simulink model "sl_quadrotorDynamics"  (R2024b)
settings: Solver=VariableStepAuto  StartTime=0.0  StopTime=50  MaxStep=0.1  RelTol=1e-3  EnableMultiTasking=on
InitFcn:
  | % load parameters of the default quadrotor
  | disp('Quadrotor parameters loaded by InitFcn')
  | mdl_quadrotor
libraries: simulink x2, roblocks x1
settings Model: Creator=corkep  LastModifiedBy=mejiasal@qut.edu.au
settings SolverCC: ZeroCrossAlgorithm=Adaptive  AlgebraicLoopSolver=TrustRegion
settings DataIOCC: LimitDataPoints=on  SaveFormat=Array  ReturnWorkspaceOutputs=off
settings OptimizationCC: BlockReduction=off  BooleanDataType=off  ReuseModelBlockBuffer=off  LifeSpan=inf
settings DebuggingCC: SaveWithParameterizedLinksMsg=none  MergeDetectMultiDrivingBlocksExec=none  SignalResolutionControl=TryResolveAllWithWarning  MaskedZcDiagnostic=none  IgnoredZcDiagnostic=none  UnconnectedInputMsg=warning  UnconnectedOutputMsg=warning  UnconnectedLineMsg=warning  SFUnexpectedBacktrackingDiag=warning  SFNoUnconditionalDefaultTransitionDiag=warning  SFExecutionAtInitializationDiag=none  ArithmeticOperatorsInVariantConditions=warning
settings HardwareCC: ProdBitPerPointer=32  ProdBitPerSizeT=32  ProdBitPerPtrDiffT=32  ProdLargestAtomicFloat=None  ProdIntDivRoundTo=Undefined  ProdEndianess=Unspecified  ProdWordSize=32  ProdHWDeviceType=32-bit Generic  TargetUnknown=on
settings ModelReferenceCC: EnableRefExpFcnMdlSchedulingChecks=on  PropagateSignalLabelsOutOfModel=off
settings SFSimCC: SimUseLocalCustomCode=off  CustomCodeUndefinedFunction=UseInterfaceOnly
settings RTWCC: RTWUseLocalCustomCode=off  GPUComputeCapability=3.5
settings CodeAppCC: StateflowObjectComments=on
settings GRTTargetCC: TargetLangStandard=C89/C90 (ANSI)
settings ConfigComp: CovMetricSettings=dw  CovSaveCumulativeToWorkspaceVar=on  CovSaveSingleToWorkspaceVar=on  CovExternalEMLEnable=off  CovSFcnEnable=off

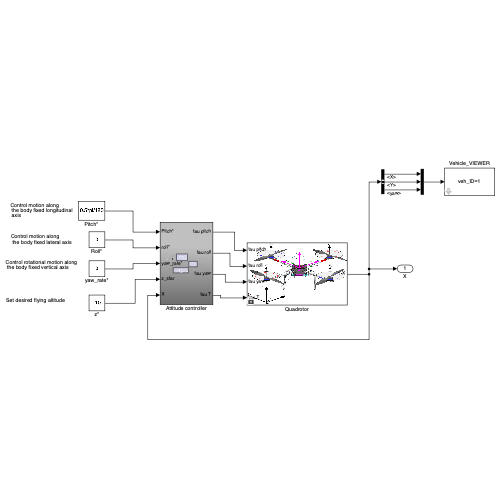
[thumbnail: Simulink's stored preview of the top-level diagram]
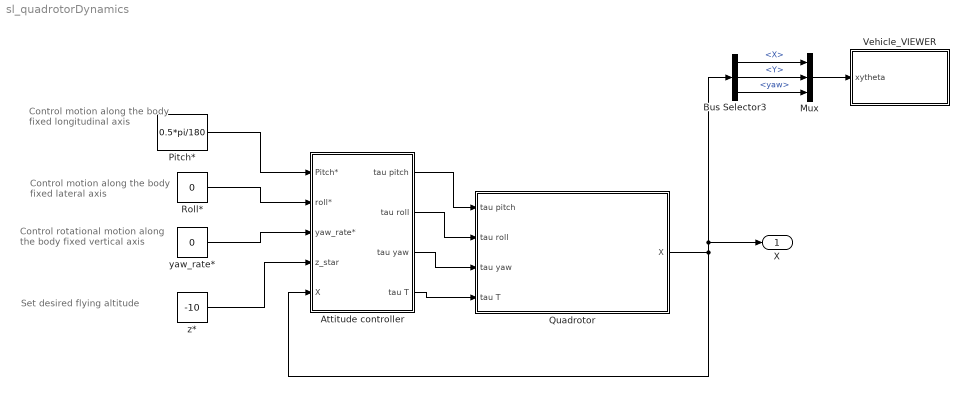
== system sl_quadrotorDynamics ==
  note: Control motion along
      |  the body fixed lateral axis
  note: Control motion along
      |  the body fixed longitudinal
      |  axis
  note: Control rotational motion along
      |  the body fixed vertical axis
  note: Set desired flying altitude
  Attitude controller : Subsystem
  Bus Selector3 : BusSelector  OutputSignals=X,Y,yaw
  Mux : Mux  Inputs=3
  Pitch* : Constant  Value=0.5*pi/180
  Quadrotor : Subsystem
      mask Display: image('quadrotor.png');
  Roll* : Constant  Value=0
  Vehicle_VIEWER : Subsystem  mask{wp_mat=[-100, 100;-100, 100]', veh_ID_num=1, veh_init_xytheta=[0 0 0], Ts=0.1}
      mask prompts: wp_mat "Waypoint matrix for arena [x_col, y_col, z_col, angle_col] (m, deg)"; veh_ID_num "Vehicle ID number"; veh_init_xytheta "Initial pose [x,y, psi]"; Ts "Sample time for updating animation (secs)"
      mask TypeOptions veh_ID_num: 1 | 2 | 3 | 4
      mask DialogControl Control2 Prompt: Animate simulation of Robot
      mask Display: fprintf('veh_ID=%d',veh_ID_num);
  yaw_rate* : Constant  Value=0
  z* : Constant  Value=-10
  X : Outport
  wires:
  Bus Selector3/1 -> Mux/1  "<X>"
  Bus Selector3/2 -> Mux/2  "<Y>"
  Bus Selector3/3 -> Mux/3  "<yaw>"
  Mux/1 -> Vehicle_VIEWER/1(xytheta)
  Roll*/1 -> Attitude controller/2(roll*)
  z*/1 -> Attitude controller/4(z_star)
  Pitch*/1 -> Attitude controller/1(Pitch*)
  yaw_rate*/1 -> Attitude controller/3(yaw_rate*)
  Quadrotor/1(X) -> X/1, Bus Selector3/1, Attitude controller/5(X)
  Attitude controller/1(tau pitch) -> Quadrotor/1(tau pitch)
  Attitude controller/2(tau roll) -> Quadrotor/2(tau roll)
  Attitude controller/3(tau yaw) -> Quadrotor/3(tau yaw)
  Attitude controller/4(tau T) -> Quadrotor/4(tau T)

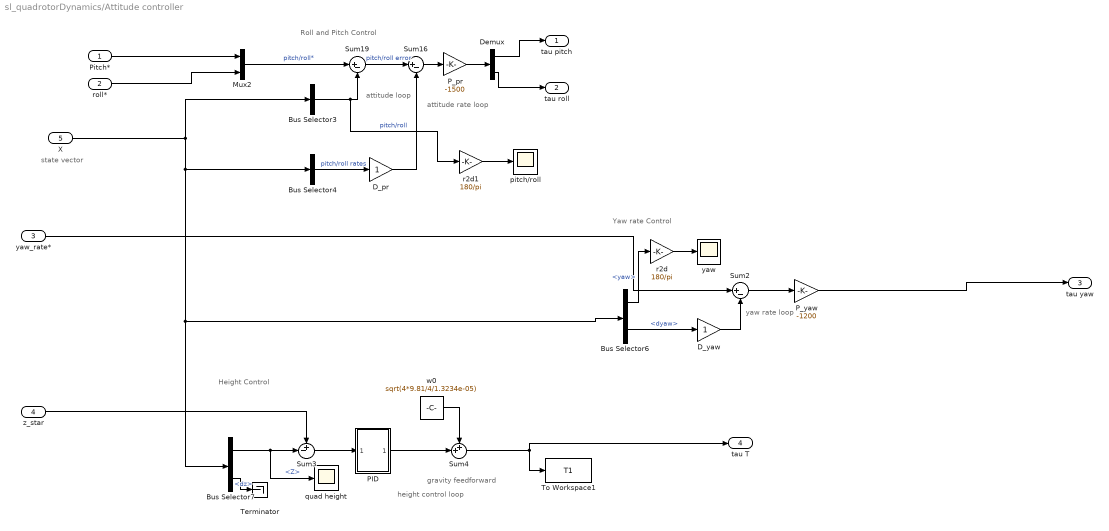
== system sl_quadrotorDynamics/Attitude controller ==
  note: Height Control
  note: Yaw rate Control
  note: Roll and Pitch Control
  note: state vector
  note: gravity feedforward
  note: attitude rate
      | loop
  note: height control
      | loop
  note: attitude
      | loop
  note: yaw rate
      | loop
  Pitch* : Inport
  roll* : Inport  Port=2
  yaw_rate* : Inport  Port=3
  z_star : Inport  Port=4
  X : Inport  Port=5
  Bus Selector3 : BusSelector  OutputSignals=pitch,roll  OutputAsBus=on
  Bus Selector4 : BusSelector  OutputSignals=dpitch,droll  OutputAsBus=on
  Bus Selector6 : BusSelector  OutputSignals=yaw,dyaw
  Bus Selector7 : BusSelector  OutputSignals=Z,dz
  D_pr : Gain
  D_yaw : Gain
  Demux : Demux  Outputs=2
  Mux2 : Mux  Inputs=2
  PID : Subsystem
  P_pr : Gain  Gain=-1500
  P_yaw : Gain  Gain=-1200
  Sum16 : Sum  Inputs=|+-
  Sum19 : Sum  Inputs=|+-
  Sum2 : Sum  Inputs=|+-
  Sum3 : Sum  Inputs=+-|
  Sum4 : Sum  Inputs=++|
  Terminator : Terminator
  To Workspace1 : ToWorkspace  VariableName=T1  SampleTime=-1
  pitch/roll : Scope
  quad height : Scope
  r2d : Gain  Gain=180/pi
  r2d1 : Gain  Gain=180/pi
  w0 : Constant  Value=sqrt(4*9.81/4/1.3234e-05)  SampleTime=0
  yaw : Scope
  tau pitch : Outport  VectorParamsAs1DForOutWhenUnconnected=off
  tau roll : Outport  Port=2  VectorParamsAs1DForOutWhenUnconnected=off
  tau yaw : Outport  Port=3  VectorParamsAs1DForOutWhenUnconnected=off
  tau T : Outport  Port=4  VectorParamsAs1DForOutWhenUnconnected=off
  wires:
  P_pr/1 -> Demux/1
  Demux/1 -> tau pitch/1
  yaw_rate*/1 -> Sum2/1
  roll*/1 -> Mux2/2
  Bus Selector6/1 -> r2d/1  "<yaw>"
  Bus Selector3/1 -> r2d1/1, Sum19/2  "pitch/roll"
  Demux/2 -> tau roll/1
  Sum16/1 -> P_pr/1
  Mux2/1 -> Sum19/1  "pitch/roll*"
  r2d/1 -> yaw/1
  z_star/1 -> Sum3/1
  Sum19/1 -> Sum16/1  "pitch/roll error"
  Pitch*/1 -> Mux2/1
  D_yaw/1 -> Sum2/2
  Bus Selector6/2 -> D_yaw/1  "<dyaw>"
  Bus Selector4/1 -> D_pr/1  "pitch/roll rates"
  Bus Selector7/1 -> quad height/1, Sum3/2  "<Z>"
  X/1 -> Bus Selector7/1, Bus Selector6/1, Bus Selector4/1, Bus Selector3/1
  Sum2/1 -> P_yaw/1
  w0/1 -> Sum4/1
  D_pr/1 -> Sum16/2
  P_yaw/1 -> tau yaw/1
  Sum4/1 -> tau T/1, To Workspace1/1
  Bus Selector7/2 -> Terminator/1  "<dz>"
  PID/1(Out1) -> Sum4/2
  Sum3/1 -> PID/1(In1)
  r2d1/1 -> pitch/roll/1

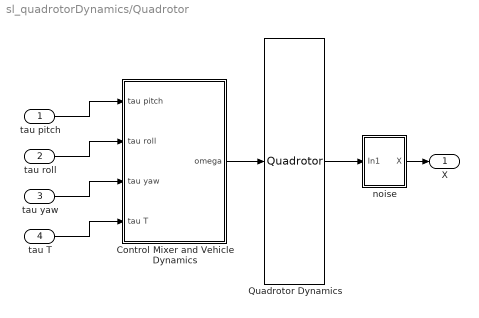
== system sl_quadrotorDynamics/Quadrotor ==
  tau pitch : Inport
  tau roll : Inport  Port=2
  tau yaw : Inport  Port=3
  tau T : Inport  Port=4
  Control Mixer and Vehicle Dynamics : Subsystem
  Quadrotor Dynamics : roblocks/Dynamics/Quadrotor  quad=quad
  noise : Subsystem
  X : Outport
  wires:
  tau yaw/1 -> Control Mixer and Vehicle Dynamics/3(tau yaw)
  tau T/1 -> Control Mixer and Vehicle Dynamics/4(tau T)
  Control Mixer and Vehicle Dynamics/1(omega) -> Quadrotor Dynamics/1
  noise/1(X) -> X/1
  tau roll/1 -> Control Mixer and Vehicle Dynamics/2(tau roll)
  tau pitch/1 -> Control Mixer and Vehicle Dynamics/1(tau pitch)
  Quadrotor Dynamics/1 -> noise/1(In1)

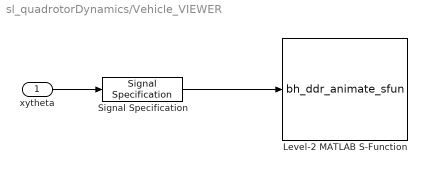
== system sl_quadrotorDynamics/Vehicle_VIEWER ==
  xytheta : Inport
  Level-2 MATLAB S-Function : M-S-Function  FunctionName=bh_ddr_animate_sfun  Parameters=Ts, wp_mat, veh_ID_num, veh_init_xytheta
  Signal Specification : SignalSpecification  Dimensions=3
  wires:
  xytheta/1 -> Signal Specification/1
  Signal Specification/1 -> Level-2 MATLAB S-Function/1

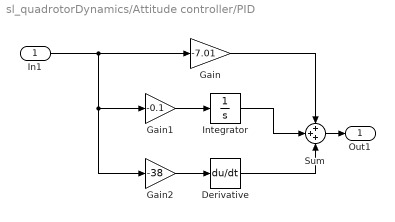
== system sl_quadrotorDynamics/Attitude controller/PID ==
  In1 : Inport
  Derivative : Derivative
  Gain : Gain  Gain=-7.01
  Gain1 : Gain  Gain=-0.1
  Gain2 : Gain  Gain=-38
  Integrator : Integrator
  Sum : Sum  Inputs=+++
  Out1 : Outport
  wires:
  Sum/1 -> Out1/1
  In1/1 -> Gain1/1, Gain2/1, Gain/1
  Gain/1 -> Sum/1
  Gain1/1 -> Integrator/1
  Integrator/1 -> Sum/2
  Gain2/1 -> Derivative/1
  Derivative/1 -> Sum/3

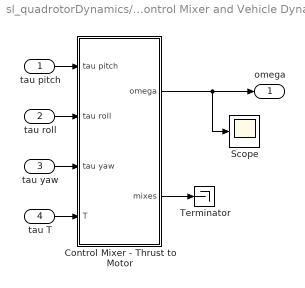
== system sl_quadrotorDynamics/Quadrotor/Control Mixer and Vehicle Dynamics ==
  tau pitch : Inport
  tau roll : Inport  Port=2
  tau yaw : Inport  Port=3
  tau T : Inport  Port=4
  Control Mixer - Thrust to Motor : Subsystem
  Scope : Scope
  Terminator : Terminator
  omega : Outport  VectorParamsAs1DForOutWhenUnconnected=off
  wires:
  Control Mixer - Thrust to Motor/2(mixes) -> Terminator/1
  tau pitch/1 -> Control Mixer - Thrust to Motor/1(tau pitch)
  tau roll/1 -> Control Mixer - Thrust to Motor/2(tau roll)
  tau yaw/1 -> Control Mixer - Thrust to Motor/3(tau yaw)
  tau T/1 -> Control Mixer - Thrust to Motor/4(T)
  Control Mixer - Thrust to Motor/1(omega) -> Scope/1, omega/1

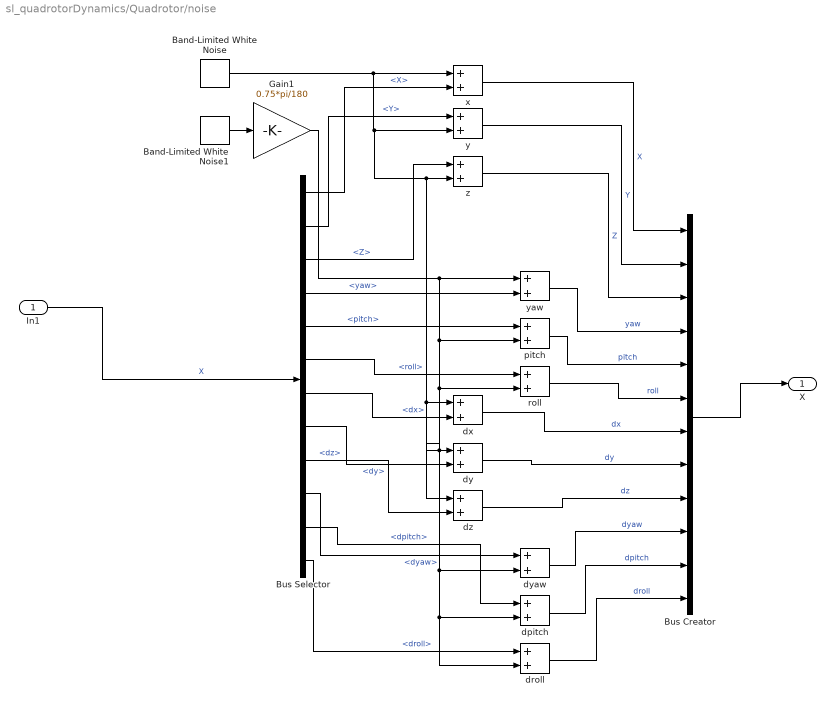
== system sl_quadrotorDynamics/Quadrotor/noise ==
  In1 : Inport
  Band-Limited White Noise : simulink/Sources/Band-Limited White Noise  Cov=[0.001]  Ts=0.1  seed=[23341]
  Band-Limited White Noise1 : simulink/Sources/Band-Limited White Noise  Cov=[0.41]  Ts=0.1  seed=[23341]
  Bus Creator : BusCreator  Inputs=12
  Bus Selector : BusSelector  OutputSignals=X,Y,Z,yaw,pitch,roll,dx,dy,dz,dyaw,dpitch,droll
  Gain1 : Gain  Gain=0.75*pi/180
  dpitch : Sum
  droll : Sum
  dx : Sum
  dy : Sum
  dyaw : Sum
  dz : Sum
  pitch : Sum
  roll : Sum
  x : Sum
  y : Sum
  yaw : Sum
  z : Sum
  X : Outport
  wires:
  x/1 -> Bus Creator/1  "X"
  Bus Selector/9 -> dz/2  "<dz>"
  Bus Selector/8 -> dy/2  "<dy>"
  Bus Selector/7 -> dx/2  "<dx>"
  y/1 -> Bus Creator/2  "Y"
  Bus Selector/6 -> roll/1  "<roll>"
  Bus Selector/5 -> pitch/1  "<pitch>"
  yaw/1 -> Bus Creator/4  "yaw"
  Bus Selector/2 -> y/1  "<Y>"
  Bus Selector/1 -> x/2  "<X>"
  Gain1/1 -> pitch/2, droll/2, dpitch/2, dyaw/2, roll/2, yaw/1
  Band-Limited White Noise/1 -> x/1, z/2, dx/1, dz/1, dy/1, y/2
  Bus Selector/10 -> dyaw/1  "<dyaw>"
  Bus Selector/11 -> dpitch/1  "<dpitch>"
  Bus Selector/4 -> yaw/2  "<yaw>"
  Bus Selector/12 -> droll/1  "<droll>"
  Band-Limited White Noise1/1 -> Gain1/1
  Bus Selector/3 -> z/1  "<Z>"
  z/1 -> Bus Creator/3  "Z"
  In1/1 -> Bus Selector/1  "X"
  Bus Creator/1 -> X/1
  pitch/1 -> Bus Creator/5  "pitch"
  roll/1 -> Bus Creator/6  "roll"
  dpitch/1 -> Bus Creator/11  "dpitch"
  droll/1 -> Bus Creator/12  "droll"
  dx/1 -> Bus Creator/7  "dx"
  dy/1 -> Bus Creator/8  "dy"
  dz/1 -> Bus Creator/9  "dz"
  dyaw/1 -> Bus Creator/10  "dyaw"

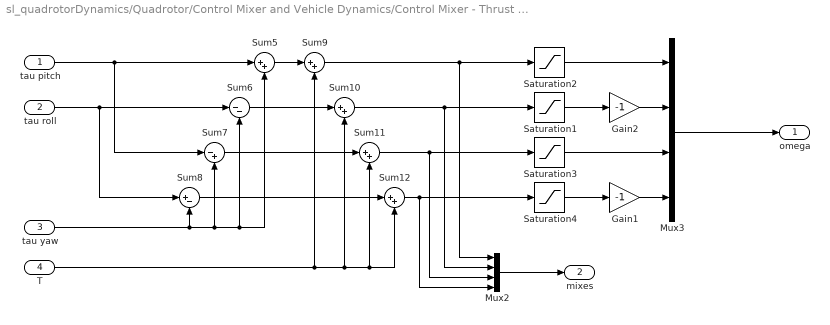
== system sl_quadrotorDynamics/Quadrotor/Control Mixer and Vehicle Dynamics/Control Mixer - Thrust to Motor ==
  tau pitch : Inport
  tau roll : Inport  Port=2
  tau yaw : Inport  Port=3
  T : Inport  Port=4
  Gain1 : Gain  Gain=-1
  Gain2 : Gain  Gain=-1
  Mux2 : Mux
  Mux3 : Mux
  Saturation{1..4} (4 alike) : Saturate  UpperLimit=1000  LowerLimit=700
  Sum{5,9..12} (5 alike) : Sum  Inputs=|++  InputSameDT=on  SaturateOnIntegerOverflow=on  OutDataTypeStr=Inherit: Same as first input
  Sum6 : Sum  Inputs=|--  InputSameDT=on  SaturateOnIntegerOverflow=on  OutDataTypeStr=Inherit: Same as first input
  Sum7 : Sum  Inputs=|-+  InputSameDT=on  SaturateOnIntegerOverflow=on  OutDataTypeStr=Inherit: Same as first input
  Sum8 : Sum  Inputs=|+-  InputSameDT=on  SaturateOnIntegerOverflow=on  OutDataTypeStr=Inherit: Same as first input
  omega : Outport  VectorParamsAs1DForOutWhenUnconnected=off
  mixes : Outport  Port=2  VectorParamsAs1DForOutWhenUnconnected=off
  wires:
  Sum7/1 -> Sum11/1
  tau roll/1 -> Sum6/1, Sum8/1
  Mux2/1 -> mixes/1
  Gain2/1 -> Mux3/2
  Sum8/1 -> Sum12/1
  Sum6/1 -> Sum10/1
  tau pitch/1 -> Sum5/1, Sum7/1
  Mux3/1 -> omega/1
  Sum10/1 -> Saturation1/1, Mux2/2
  Sum12/1 -> Saturation4/1, Mux2/4
  Saturation1/1 -> Gain2/1
  Saturation3/1 -> Mux3/3
  T/1 -> Sum11/2, Sum12/2, Sum10/2, Sum9/2
  tau yaw/1 -> Sum8/2, Sum7/2, Sum6/2, Sum5/2
  Saturation4/1 -> Gain1/1
  Sum9/1 -> Saturation2/1, Mux2/1
  Sum11/1 -> Saturation3/1, Mux2/3
  Saturation2/1 -> Mux3/1
  Sum5/1 -> Sum9/1
  Gain1/1 -> Mux3/4
